simulink model "SOP_tester"  (R2024a)
settings: Solver=VariableStepAuto  StartTime=0.0  StopTime=stop_time  RelTol=1e-3
settings Model: DataDictionary=SOP_dictionary.sldd  Creator=mmackenzie  LastModifiedBy=mmackenzie
settings OptimizationCC: ReuseModelBlockBuffer=off
settings RTWCC: GPUComputeCapability=3.5

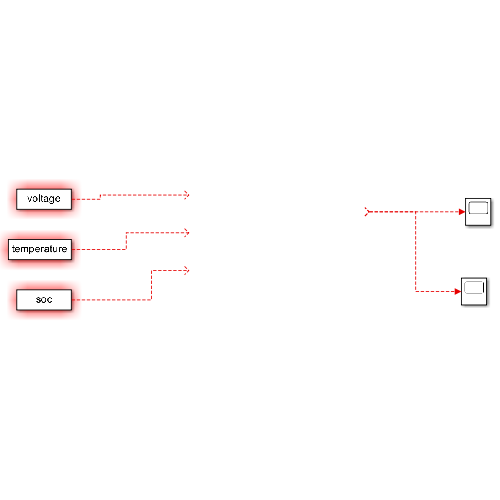
[thumbnail: Simulink's stored preview of the top-level diagram]
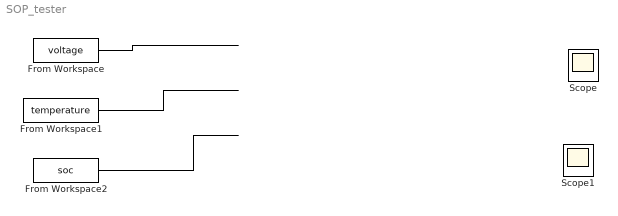
== system SOP_tester ==
  From Workspace : FromWorkspace  VariableName=voltage
  From Workspace1 : FromWorkspace  VariableName=temperature
  From Workspace2 : FromWorkspace  VariableName=soc
  Scope : Scope
  Scope1 : Scope
  wires:
  From Workspace/1 -> ?
  From Workspace1/1 -> ?
  From Workspace2/1 -> ?
  ? -> Scope/1
  ? -> Scope1/1
